simulink model "Racing_Mode"  (R2017b)
settings: Solver=FixedStepAuto  StartTime=0.0  StopTime=10.0  RelTol=1e-3
libraries: simulink x1
settings Model: Creator=cspt  LastModifiedBy=joanv
settings RTWCC: SystemTargetFile=irt.tlc  TemplateMakefile=irt_default_tmf  Description=INTECRIO Real-Time Target
settings STFCustomTargetCC: TargetLangStandard=C99 (ISO)  UtilityFuncGeneration=Shared location  SystemTargetFile=irt.tlc
settings GRTTargetCC: UtilityFuncGeneration=Shared location  ParMdlRefBuildCompliant=off  CompOptLevelCompliant=off  ConcurrentExecutionCompliant=off  CombineOutputUpdateFcns=off  MatFileLogging=off  CPPClassGenCompliant=off  GRTInterface=on  UseToolchainInfoCompliant=off  GenerateASAP2=on

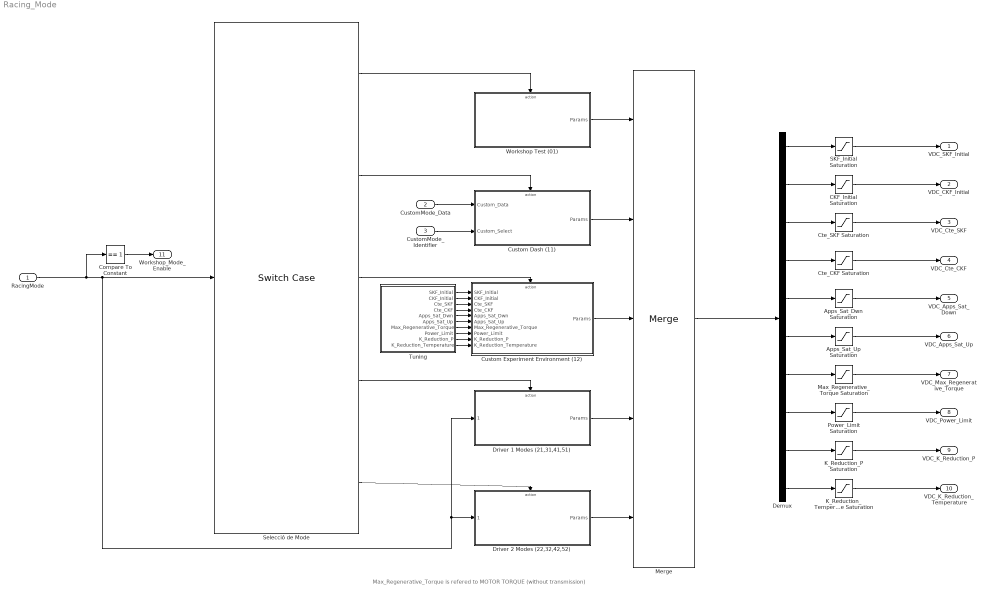
== system Racing_Mode ==
  note: Max_Regenerative_Torque is refered to MOTOR TORQUE (without transmission)
  RacingMode : Inport  OutDataTypeStr=uint8
  CustomMode_Data : Inport  Port=2
  CustomMode_Identifier : Inport  Port=3
  Apps_Sat_Dwn Saturation : Saturate  LowerLimit=0
  Apps_Sat_Up Saturation : Saturate  UpperLimit=1  LowerLimit=0
  CKF_Initial Saturation : Saturate  UpperLimit=0.9  LowerLimit=0
  Compare To Constant : simulink/Logic and Bit Operations/Compare To Constant  relop===  const=1  OutDataTypeStr=boolean
  Cte_CKF Saturation : Saturate  UpperLimit=1  LowerLimit=0
  Cte_SKF Saturation : Saturate  UpperLimit=1  LowerLimit=0
  Custom Dash (11) : Subsystem  TreatAsAtomicUnit=on
  Custom Experiment Environment (12) : Subsystem  TreatAsAtomicUnit=on
  Demux : Demux  Outputs=10
  Driver 1 Modes (21,31,41,51) : Subsystem  TreatAsAtomicUnit=on
  Driver 2 Modes (22,32,42,52) : Subsystem  TreatAsAtomicUnit=on
  K_Reduction_P Saturation : Saturate  UpperLimit=1  LowerLimit=0
  K_Reduction_Temperature Saturation : Saturate  UpperLimit=1  LowerLimit=0
  Max_Regenerative_Torque Saturation : Saturate  UpperLimit=10  LowerLimit=0
  Merge : Merge  Inputs=5
  Power_Limit Saturation : Saturate  UpperLimit=77  LowerLimit=0
  SKF_Initial Saturation : Saturate  UpperLimit=0.9  LowerLimit=0
  Selecció de Mode : SwitchCase  CaseConditions={01, 11, 12, [21,31,41,51], [22,32,42,52]}  ShowDefaultCase=off
  Tuning : Subsystem
  Workshop Test (01) : Subsystem  TreatAsAtomicUnit=on
  VDC_SKF_Initial : Outport
  VDC_CKF_Initial : Outport  Port=2
  VDC_Cte_SKF : Outport  Port=3
  VDC_Cte_CKF : Outport  Port=4
  VDC_Apps_Sat_Down : Outport  Port=5
  VDC_Apps_Sat_Up : Outport  Port=6
  VDC_Max_Regenerative_Torque : Outport  Port=7
  VDC_Power_Limit : Outport  Port=8
  VDC_K_Reduction_P : Outport  Port=9
  VDC_K_Reduction_Temperature : Outport  Port=10
  Workshop_Mode_Enable : Outport  Port=11
  wires:
  RacingMode/1 -> Compare To Constant/1, Driver 2 Modes (22,32,42,52)/1(" "), Driver 1 Modes (21,31,41,51)/1(" "), Selecció de Mode/1
  CKF_Initial Saturation/1 -> VDC_CKF_Initial/1
  Demux/6 -> Apps_Sat_Up Saturation/1
  Demux/3 -> Cte_SKF Saturation/1
  Demux/2 -> CKF_Initial Saturation/1
  Power_Limit Saturation/1 -> VDC_Power_Limit/1
  Apps_Sat_Up Saturation/1 -> VDC_Apps_Sat_Up/1
  Merge/1 -> Demux/1
  CustomMode_Data/1 -> Custom Dash (11)/1(Custom_Data)
  Tuning/7(Max_Regenerative_Torque) -> Custom Experiment Environment (12)/7(Max_Regenerative_Torque)
  Custom Experiment Environment (12)/1(Params) -> Merge/3
  Tuning/9(K_Reduction_P) -> Custom Experiment Environment (12)/9(K_Reduction_P)
  Demux/8 -> Power_Limit Saturation/1
  Tuning/8(Power_Limit) -> Custom Experiment Environment (12)/8(Power_Limit)
  Tuning/4(Cte_CKF) -> Custom Experiment Environment (12)/4(Cte_CKF)
  Selecció de Mode/4 -> Driver 1 Modes (21,31,41,51)/Action
  Demux/4 -> Cte_CKF Saturation/1
  K_Reduction_Temperature Saturation/1 -> VDC_K_Reduction_Temperature/1
  Selecció de Mode/2 -> Custom Dash (11)/Action
  Selecció de Mode/1 -> Workshop Test (01)/Action
  Demux/9 -> K_Reduction_P Saturation/1
  Demux/10 -> K_Reduction_Temperature Saturation/1
  Workshop Test (01)/1(Params) -> Merge/1
  Tuning/5(Apps_Sat_Dwn) -> Custom Experiment Environment (12)/5(Apps_Sat_Dwn)
  Selecció de Mode/5 -> Driver 2 Modes (22,32,42,52)/Action
  Max_Regenerative_Torque Saturation/1 -> VDC_Max_Regenerative_Torque/1
  Cte_CKF Saturation/1 -> VDC_Cte_CKF/1
  Driver 2 Modes (22,32,42,52)/1(Params) -> Merge/5
  Apps_Sat_Dwn Saturation/1 -> VDC_Apps_Sat_Down/1
  Tuning/3(Cte_SKF) -> Custom Experiment Environment (12)/3(Cte_SKF)
  Cte_SKF Saturation/1 -> VDC_Cte_SKF/1
  Tuning/6(Apps_Sat_Up) -> Custom Experiment Environment (12)/6(Apps_Sat_Up)
  Tuning/2(CKF_Initial) -> Custom Experiment Environment (12)/2(CKF_Initial)
  Demux/1 -> SKF_Initial Saturation/1
  K_Reduction_P Saturation/1 -> VDC_K_Reduction_P/1
  Custom Dash (11)/1(Params) -> Merge/2
  Demux/7 -> Max_Regenerative_Torque Saturation/1
  Selecció de Mode/3 -> Custom Experiment Environment (12)/Action
  Tuning/10(K_Reduction_Temperature) -> Custom Experiment Environment (12)/10(K_Reduction_Temperature)
  Demux/5 -> Apps_Sat_Dwn Saturation/1
  SKF_Initial Saturation/1 -> VDC_SKF_Initial/1
  Tuning/1(SKF_Initial) -> Custom Experiment Environment (12)/1(SKF_Initial)
  Driver 1 Modes (21,31,41,51)/1(Params) -> Merge/4
  CustomMode_Identifier/1 -> Custom Dash (11)/2(Custom_Select)
  Compare To Constant/1 -> Workshop_Mode_Enable/1

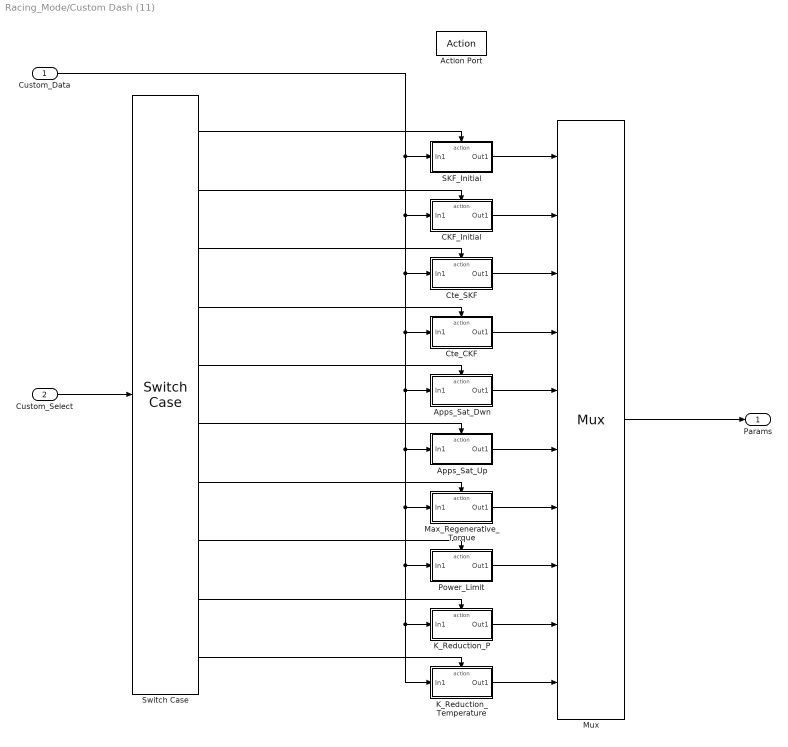
== system Racing_Mode/Custom Dash (11) ==
  Custom_Data : Inport
  Custom_Select : Inport  Port=2
  Action Port : ActionPort  ActionType=case
  Apps_Sat_Dwn : Subsystem  TreatAsAtomicUnit=on
  Apps_Sat_Up : Subsystem  TreatAsAtomicUnit=on
  CKF_Initial : Subsystem  TreatAsAtomicUnit=on
  Cte_CKF : Subsystem  TreatAsAtomicUnit=on
  Cte_SKF : Subsystem  TreatAsAtomicUnit=on
  K_Reduction_P : Subsystem  TreatAsAtomicUnit=on
  K_Reduction_Temperature : Subsystem  TreatAsAtomicUnit=on
  Max_Regenerative_Torque : Subsystem  TreatAsAtomicUnit=on
  Mux : Mux  Inputs=10
  Power_Limit : Subsystem  TreatAsAtomicUnit=on
  SKF_Initial : Subsystem  TreatAsAtomicUnit=on
  Switch Case : SwitchCase  CaseConditions={1,2,3,4,5,6,7,8,9,10}  ShowDefaultCase=off
  Params : Outport
  wires:
  Custom_Select/1 -> Switch Case/1
  Custom_Data/1 -> K_Reduction_Temperature/1(In1), K_Reduction_P/1(In1), Power_Limit/1(In1), Max_Regenerative_Torque/1(In1), Apps_Sat_Up/1(In1), Apps_Sat_Dwn/1(In1), Cte_CKF/1(In1), Cte_SKF/1(In1), CKF_Initial/1(In1), SKF_Initial/1(In1)
  Switch Case/1 -> SKF_Initial/Action
  SKF_Initial/1(Out1) -> Mux/1
  Mux/1 -> Params/1
  CKF_Initial/1(Out1) -> Mux/2
  Cte_SKF/1(Out1) -> Mux/3
  Cte_CKF/1(Out1) -> Mux/4
  Apps_Sat_Dwn/1(Out1) -> Mux/5
  Apps_Sat_Up/1(Out1) -> Mux/6
  Max_Regenerative_Torque/1(Out1) -> Mux/7
  Power_Limit/1(Out1) -> Mux/8
  K_Reduction_P/1(Out1) -> Mux/9
  K_Reduction_Temperature/1(Out1) -> Mux/10
  Switch Case/2 -> CKF_Initial/Action
  Switch Case/3 -> Cte_SKF/Action
  Switch Case/4 -> Cte_CKF/Action
  Switch Case/5 -> Apps_Sat_Dwn/Action
  Switch Case/6 -> Apps_Sat_Up/Action
  Switch Case/7 -> Max_Regenerative_Torque/Action
  Switch Case/8 -> Power_Limit/Action
  Switch Case/9 -> K_Reduction_P/Action
  Switch Case/10 -> K_Reduction_Temperature/Action

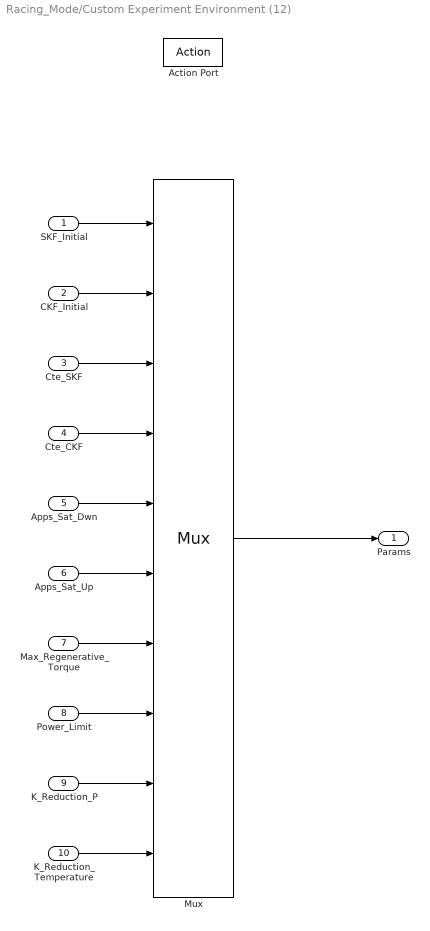
== system Racing_Mode/Custom Experiment Environment (12) ==
  SKF_Initial : Inport
  CKF_Initial : Inport  Port=2
  Cte_SKF : Inport  Port=3
  Cte_CKF : Inport  Port=4
  Apps_Sat_Dwn : Inport  Port=5
  Apps_Sat_Up : Inport  Port=6
  Max_Regenerative_Torque : Inport  Port=7
  Power_Limit : Inport  Port=8
  K_Reduction_P : Inport  Port=9
  K_Reduction_Temperature : Inport  Port=10
  Action Port : ActionPort  ActionType=case
  Mux : Mux  Inputs=10
  Params : Outport
  wires:
  Mux/1 -> Params/1
  K_Reduction_Temperature/1 -> Mux/10
  K_Reduction_P/1 -> Mux/9
  Power_Limit/1 -> Mux/8
  Max_Regenerative_Torque/1 -> Mux/7
  Apps_Sat_Up/1 -> Mux/6
  Apps_Sat_Dwn/1 -> Mux/5
  Cte_CKF/1 -> Mux/4
  Cte_SKF/1 -> Mux/3
  CKF_Initial/1 -> Mux/2
  SKF_Initial/1 -> Mux/1

== system Racing_Mode/Driver 1 Modes (21,31,41,51) ==
  " " : Inport  OutDataTypeStr=uint8
  Action Port : ActionPort  ActionType=case
  "Acceleration (2). Driver 1 (1) " : Subsystem  TreatAsAtomicUnit=on
  AutoX (4). Driver 1 (1) : Subsystem  TreatAsAtomicUnit=on
  Endurance (5). Driver 1 (1) : Subsystem  TreatAsAtomicUnit=on
  Merge : Merge  Inputs=4
  Selecció de Mode : SwitchCase  CaseConditions={21,31,41,51}  ShowDefaultCase=off
  Skidpad (3). Driver 1 (1) : Subsystem  TreatAsAtomicUnit=on
  Params : Outport
  wires:
  Merge/1 -> Params/1
  " "/1 -> Selecció de Mode/1
  Selecció de Mode/4 -> Endurance (5). Driver 1 (1)/Action
  Selecció de Mode/3 -> AutoX (4). Driver 1 (1)/Action
  Selecció de Mode/2 -> Skidpad (3). Driver 1 (1)/Action
  Selecció de Mode/1 -> "Acceleration (2). Driver 1 (1) "/Action
  "Acceleration (2). Driver 1 (1) "/1(Params) -> Merge/1
  Skidpad (3). Driver 1 (1)/1(Params) -> Merge/2
  AutoX (4). Driver 1 (1)/1(Params) -> Merge/3
  Endurance (5). Driver 1 (1)/1(Params) -> Merge/4

== system Racing_Mode/Driver 2 Modes (22,32,42,52) ==
  " " : Inport  OutDataTypeStr=uint8
  Action Port : ActionPort  ActionType=case
  "Acceleration (2). Driver 2 (2) " : Subsystem  TreatAsAtomicUnit=on
  AutoX (4). Driver 2 (2) : Subsystem  TreatAsAtomicUnit=on
  Endurance (5). Driver 2 (2) : Subsystem  TreatAsAtomicUnit=on
  Merge : Merge  Inputs=4
  Selecció de Mode : SwitchCase  CaseConditions={22,32,42,52}  ShowDefaultCase=off
  Skidpad (3). Driver 2 (2) : Subsystem  TreatAsAtomicUnit=on
  Params : Outport
  wires:
  Merge/1 -> Params/1
  " "/1 -> Selecció de Mode/1
  "Acceleration (2). Driver 2 (2) "/1(Params) -> Merge/1
  Skidpad (3). Driver 2 (2)/1(Params) -> Merge/2
  AutoX (4). Driver 2 (2)/1(Params) -> Merge/3
  Endurance (5). Driver 2 (2)/1(Params) -> Merge/4
  Selecció de Mode/4 -> Endurance (5). Driver 2 (2)/Action
  Selecció de Mode/3 -> AutoX (4). Driver 2 (2)/Action
  Selecció de Mode/2 -> Skidpad (3). Driver 2 (2)/Action
  Selecció de Mode/1 -> "Acceleration (2). Driver 2 (2) "/Action

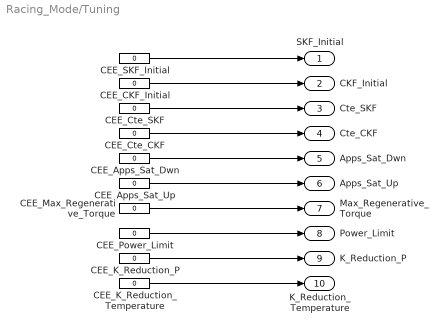
== system Racing_Mode/Tuning ==
  CEE_Apps_Sat_Dwn : Constant  Value=0
  CEE_Apps_Sat_Up : Constant  Value=0
  CEE_CKF_Initial : Constant  Value=0
  CEE_Cte_CKF : Constant  Value=0
  CEE_Cte_SKF : Constant  Value=0
  CEE_K_Reduction_P : Constant  Value=0
  CEE_K_Reduction_Temperature : Constant  Value=0
  CEE_Max_Regenerative_Torque : Constant  Value=0
  CEE_Power_Limit : Constant  Value=0
  CEE_SKF_Initial : Constant  Value=0
  SKF_Initial : Outport
  CKF_Initial : Outport  Port=2
  Cte_SKF : Outport  Port=3
  Cte_CKF : Outport  Port=4
  Apps_Sat_Dwn : Outport  Port=5
  Apps_Sat_Up : Outport  Port=6
  Max_Regenerative_Torque : Outport  Port=7
  Power_Limit : Outport  Port=8
  K_Reduction_P : Outport  Port=9
  K_Reduction_Temperature : Outport  Port=10
  wires:
  CEE_Cte_SKF/1 -> Cte_SKF/1
  CEE_CKF_Initial/1 -> CKF_Initial/1
  CEE_Apps_Sat_Dwn/1 -> Apps_Sat_Dwn/1
  CEE_SKF_Initial/1 -> SKF_Initial/1
  CEE_Max_Regenerative_Torque/1 -> Max_Regenerative_Torque/1
  CEE_Power_Limit/1 -> Power_Limit/1
  CEE_K_Reduction_P/1 -> K_Reduction_P/1
  CEE_K_Reduction_Temperature/1 -> K_Reduction_Temperature/1
  CEE_Apps_Sat_Up/1 -> Apps_Sat_Up/1
  CEE_Cte_CKF/1 -> Cte_CKF/1

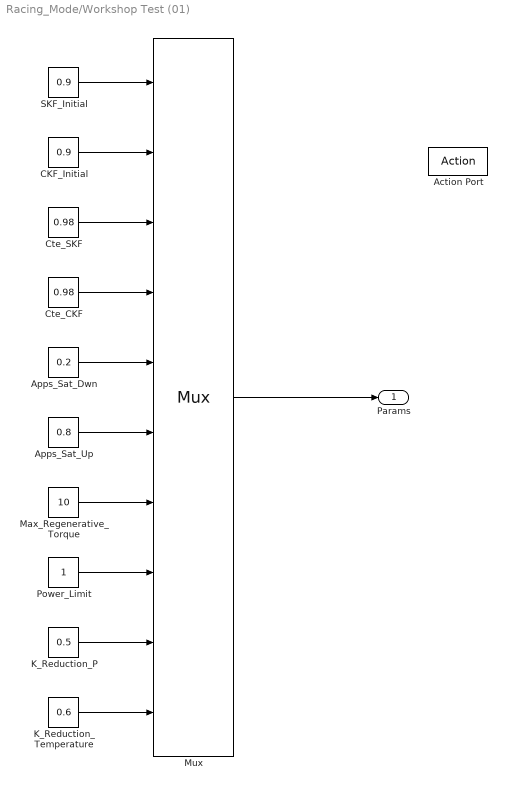
== system Racing_Mode/Workshop Test (01) ==
  Action Port : ActionPort  ActionType=case
  Apps_Sat_Dwn : Constant  Value=0.2
  Apps_Sat_Up : Constant  Value=0.8
  CKF_Initial : Constant  Value=0.9
  Cte_CKF : Constant  Value=0.98
  Cte_SKF : Constant  Value=0.98
  K_Reduction_P : Constant  Value=0.5
  K_Reduction_Temperature : Constant  Value=0.6
  Max_Regenerative_Torque : Constant  Value=10
  Mux : Mux  Inputs=10
  Power_Limit : Constant
  SKF_Initial : Constant  Value=0.9
  Params : Outport
  wires:
  Mux/1 -> Params/1
  SKF_Initial/1 -> Mux/1
  Cte_SKF/1 -> Mux/3
  CKF_Initial/1 -> Mux/2
  Cte_CKF/1 -> Mux/4
  Apps_Sat_Dwn/1 -> Mux/5
  Apps_Sat_Up/1 -> Mux/6
  K_Reduction_Temperature/1 -> Mux/10
  K_Reduction_P/1 -> Mux/9
  Power_Limit/1 -> Mux/8
  Max_Regenerative_Torque/1 -> Mux/7

== system Racing_Mode/Custom Dash (11)/Apps_Sat_Dwn ==
  In1 : Inport
  Action Port : ActionPort  ActionType=case
  Gain : Gain  Gain=1/100
  Out1 : Outport
  wires:
  In1/1 -> Gain/1
  Gain/1 -> Out1/1

== system Racing_Mode/Custom Dash (11)/Apps_Sat_Up ==
  In1 : Inport
  Action Port : ActionPort  ActionType=case
  Gain : Gain  Gain=1/100
  Out1 : Outport
  wires:
  In1/1 -> Gain/1
  Gain/1 -> Out1/1

== system Racing_Mode/Custom Dash (11)/CKF_Initial ==
  In1 : Inport
  Action Port : ActionPort  ActionType=case
  Gain : Gain  Gain=1/1000
  Out1 : Outport
  wires:
  In1/1 -> Gain/1
  Gain/1 -> Out1/1

== system Racing_Mode/Custom Dash (11)/Cte_CKF ==
  In1 : Inport
  Action Port : ActionPort  ActionType=case
  Gain : Gain  Gain=1/1000
  Out1 : Outport
  wires:
  In1/1 -> Gain/1
  Gain/1 -> Out1/1

== system Racing_Mode/Custom Dash (11)/Cte_SKF ==
  In1 : Inport
  Action Port : ActionPort  ActionType=case
  Gain : Gain  Gain=1/1000
  Out1 : Outport
  wires:
  In1/1 -> Gain/1
  Gain/1 -> Out1/1

== system Racing_Mode/Custom Dash (11)/K_Reduction_P ==
  In1 : Inport
  Action Port : ActionPort  ActionType=case
  Gain : Gain  Gain=1/100
  Out1 : Outport
  wires:
  In1/1 -> Gain/1
  Gain/1 -> Out1/1

== system Racing_Mode/Custom Dash (11)/K_Reduction_Temperature ==
  In1 : Inport
  Action Port : ActionPort  ActionType=case
  Gain : Gain  Gain=1/100
  Out1 : Outport
  wires:
  In1/1 -> Gain/1
  Gain/1 -> Out1/1

== system Racing_Mode/Custom Dash (11)/Max_Regenerative_Torque ==
  In1 : Inport
  Action Port : ActionPort  ActionType=case
  Out1 : Outport
  wires:
  In1/1 -> Out1/1

== system Racing_Mode/Custom Dash (11)/Power_Limit ==
  In1 : Inport
  Action Port : ActionPort  ActionType=case
  Out1 : Outport
  wires:
  In1/1 -> Out1/1

== system Racing_Mode/Custom Dash (11)/SKF_Initial ==
  In1 : Inport
  Action Port : ActionPort  ActionType=case
  Gain : Gain  Gain=1/1000
  Out1 : Outport
  wires:
  In1/1 -> Gain/1
  Gain/1 -> Out1/1

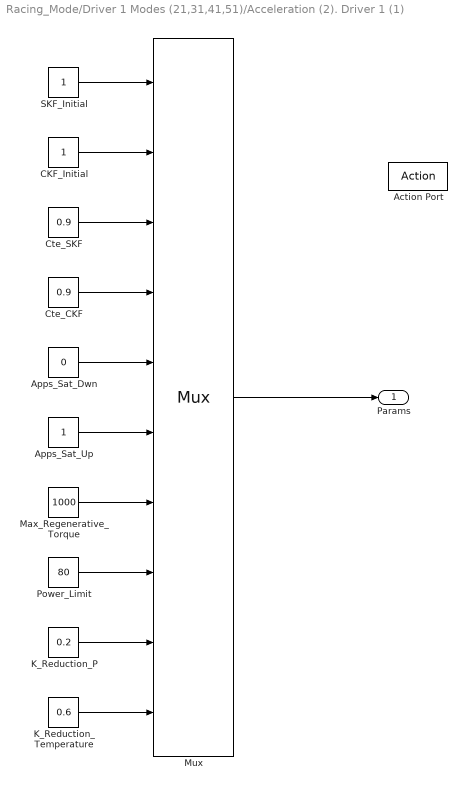
== system Racing_Mode/Driver 1 Modes (21,31,41,51)/Acceleration (2). Driver 1 (1)  ==
  Action Port : ActionPort  ActionType=case
  Apps_Sat_Dwn : Constant  Value=0
  Apps_Sat_Up : Constant
  CKF_Initial : Constant
  Cte_CKF : Constant  Value=0.9
  Cte_SKF : Constant  Value=0.9
  K_Reduction_P : Constant  Value=0.2
  K_Reduction_Temperature : Constant  Value=0.6
  Max_Regenerative_Torque : Constant  Value=1000
  Mux : Mux  Inputs=10
  Power_Limit : Constant  Value=80
  SKF_Initial : Constant
  Params : Outport
  wires:
  Mux/1 -> Params/1
  SKF_Initial/1 -> Mux/1
  Cte_SKF/1 -> Mux/3
  CKF_Initial/1 -> Mux/2
  Cte_CKF/1 -> Mux/4
  Apps_Sat_Dwn/1 -> Mux/5
  Apps_Sat_Up/1 -> Mux/6
  K_Reduction_Temperature/1 -> Mux/10
  K_Reduction_P/1 -> Mux/9
  Power_Limit/1 -> Mux/8
  Max_Regenerative_Torque/1 -> Mux/7

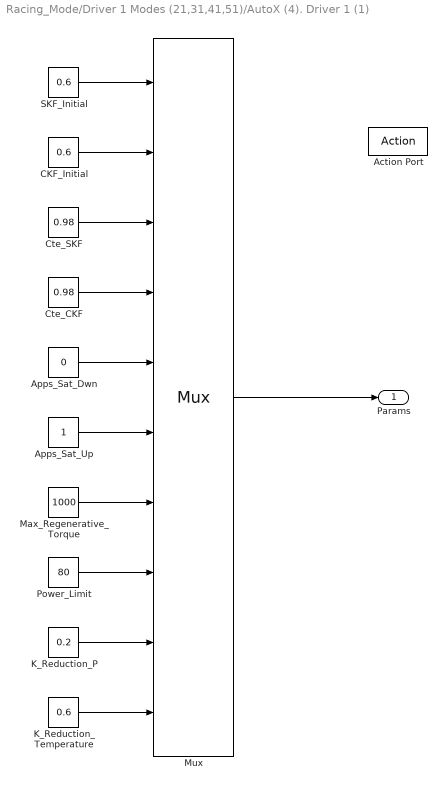
== system Racing_Mode/Driver 1 Modes (21,31,41,51)/AutoX (4). Driver 1 (1) ==
  Action Port : ActionPort  ActionType=case
  Apps_Sat_Dwn : Constant  Value=0
  Apps_Sat_Up : Constant
  CKF_Initial : Constant  Value=0.6
  Cte_CKF : Constant  Value=0.98
  Cte_SKF : Constant  Value=0.98
  K_Reduction_P : Constant  Value=0.2
  K_Reduction_Temperature : Constant  Value=0.6
  Max_Regenerative_Torque : Constant  Value=1000
  Mux : Mux  Inputs=10
  Power_Limit : Constant  Value=80
  SKF_Initial : Constant  Value=0.6
  Params : Outport
  wires:
  Mux/1 -> Params/1
  SKF_Initial/1 -> Mux/1
  Cte_SKF/1 -> Mux/3
  CKF_Initial/1 -> Mux/2
  Cte_CKF/1 -> Mux/4
  Apps_Sat_Dwn/1 -> Mux/5
  Apps_Sat_Up/1 -> Mux/6
  K_Reduction_Temperature/1 -> Mux/10
  K_Reduction_P/1 -> Mux/9
  Power_Limit/1 -> Mux/8
  Max_Regenerative_Torque/1 -> Mux/7

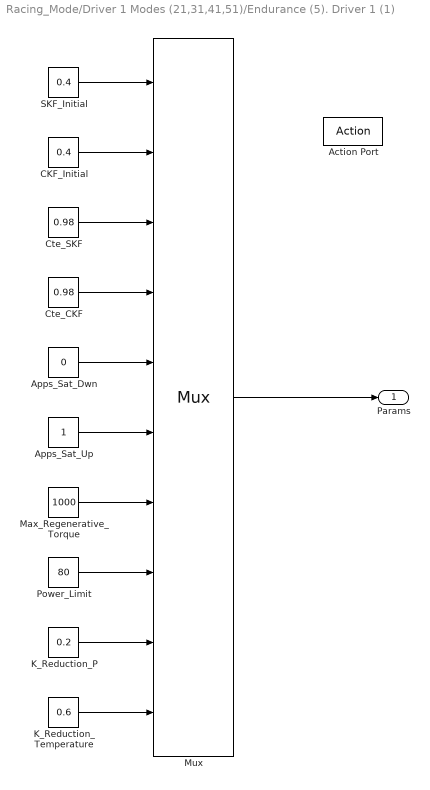
== system Racing_Mode/Driver 1 Modes (21,31,41,51)/Endurance (5). Driver 1 (1) ==
  Action Port : ActionPort  ActionType=case
  Apps_Sat_Dwn : Constant  Value=0
  Apps_Sat_Up : Constant
  CKF_Initial : Constant  Value=0.4
  Cte_CKF : Constant  Value=0.98
  Cte_SKF : Constant  Value=0.98
  K_Reduction_P : Constant  Value=0.2
  K_Reduction_Temperature : Constant  Value=0.6
  Max_Regenerative_Torque : Constant  Value=1000
  Mux : Mux  Inputs=10
  Power_Limit : Constant  Value=80
  SKF_Initial : Constant  Value=0.4
  Params : Outport
  wires:
  Mux/1 -> Params/1
  SKF_Initial/1 -> Mux/1
  Cte_SKF/1 -> Mux/3
  CKF_Initial/1 -> Mux/2
  Cte_CKF/1 -> Mux/4
  Apps_Sat_Dwn/1 -> Mux/5
  Apps_Sat_Up/1 -> Mux/6
  K_Reduction_Temperature/1 -> Mux/10
  K_Reduction_P/1 -> Mux/9
  Power_Limit/1 -> Mux/8
  Max_Regenerative_Torque/1 -> Mux/7

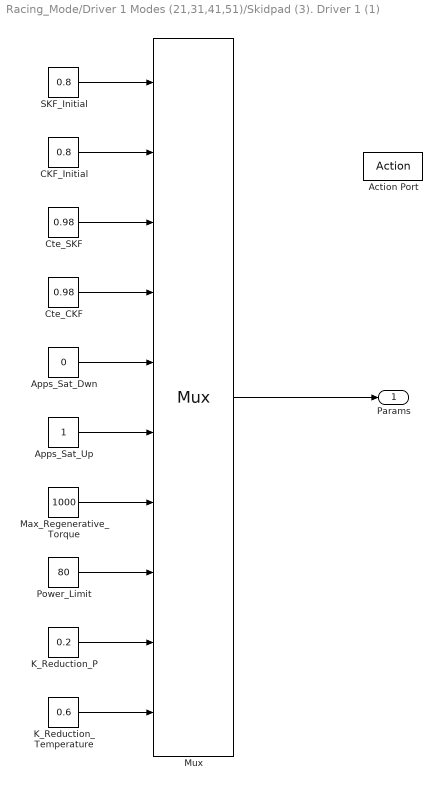
== system Racing_Mode/Driver 1 Modes (21,31,41,51)/Skidpad (3). Driver 1 (1) ==
  Action Port : ActionPort  ActionType=case
  Apps_Sat_Dwn : Constant  Value=0
  Apps_Sat_Up : Constant
  CKF_Initial : Constant  Value=0.8
  Cte_CKF : Constant  Value=0.98
  Cte_SKF : Constant  Value=0.98
  K_Reduction_P : Constant  Value=0.2
  K_Reduction_Temperature : Constant  Value=0.6
  Max_Regenerative_Torque : Constant  Value=1000
  Mux : Mux  Inputs=10
  Power_Limit : Constant  Value=80
  SKF_Initial : Constant  Value=0.8
  Params : Outport
  wires:
  Mux/1 -> Params/1
  SKF_Initial/1 -> Mux/1
  Cte_SKF/1 -> Mux/3
  CKF_Initial/1 -> Mux/2
  Cte_CKF/1 -> Mux/4
  Apps_Sat_Dwn/1 -> Mux/5
  Apps_Sat_Up/1 -> Mux/6
  K_Reduction_Temperature/1 -> Mux/10
  K_Reduction_P/1 -> Mux/9
  Power_Limit/1 -> Mux/8
  Max_Regenerative_Torque/1 -> Mux/7

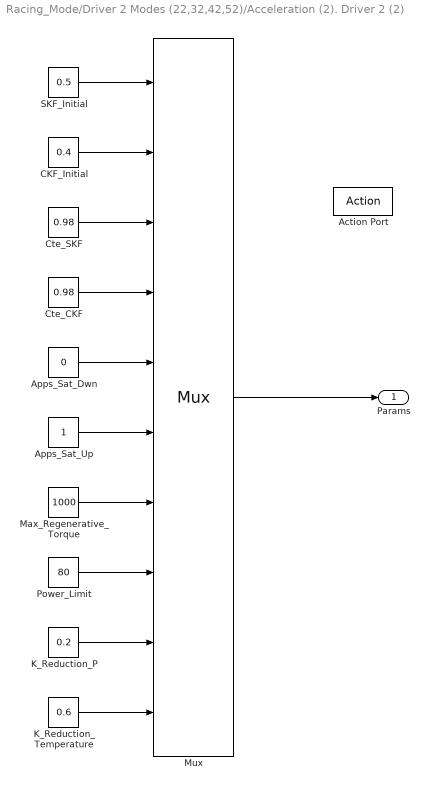
== system Racing_Mode/Driver 2 Modes (22,32,42,52)/Acceleration (2). Driver 2 (2)  ==
  Action Port : ActionPort  ActionType=case
  Apps_Sat_Dwn : Constant  Value=0
  Apps_Sat_Up : Constant
  CKF_Initial : Constant  Value=0.4
  Cte_CKF : Constant  Value=0.98
  Cte_SKF : Constant  Value=0.98
  K_Reduction_P : Constant  Value=0.2
  K_Reduction_Temperature : Constant  Value=0.6
  Max_Regenerative_Torque : Constant  Value=1000
  Mux : Mux  Inputs=10
  Power_Limit : Constant  Value=80
  SKF_Initial : Constant  Value=0.5
  Params : Outport
  wires:
  Mux/1 -> Params/1
  SKF_Initial/1 -> Mux/1
  Cte_SKF/1 -> Mux/3
  CKF_Initial/1 -> Mux/2
  Cte_CKF/1 -> Mux/4
  Apps_Sat_Dwn/1 -> Mux/5
  Apps_Sat_Up/1 -> Mux/6
  K_Reduction_Temperature/1 -> Mux/10
  K_Reduction_P/1 -> Mux/9
  Power_Limit/1 -> Mux/8
  Max_Regenerative_Torque/1 -> Mux/7

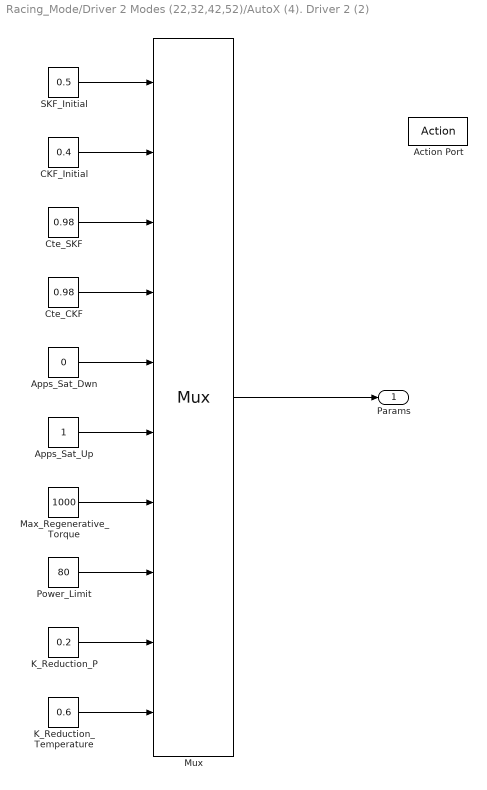
== system Racing_Mode/Driver 2 Modes (22,32,42,52)/AutoX (4). Driver 2 (2) ==
  Action Port : ActionPort  ActionType=case
  Apps_Sat_Dwn : Constant  Value=0
  Apps_Sat_Up : Constant
  CKF_Initial : Constant  Value=0.4
  Cte_CKF : Constant  Value=0.98
  Cte_SKF : Constant  Value=0.98
  K_Reduction_P : Constant  Value=0.2
  K_Reduction_Temperature : Constant  Value=0.6
  Max_Regenerative_Torque : Constant  Value=1000
  Mux : Mux  Inputs=10
  Power_Limit : Constant  Value=80
  SKF_Initial : Constant  Value=0.5
  Params : Outport
  wires:
  Mux/1 -> Params/1
  SKF_Initial/1 -> Mux/1
  Cte_SKF/1 -> Mux/3
  CKF_Initial/1 -> Mux/2
  Cte_CKF/1 -> Mux/4
  Apps_Sat_Dwn/1 -> Mux/5
  Apps_Sat_Up/1 -> Mux/6
  K_Reduction_Temperature/1 -> Mux/10
  K_Reduction_P/1 -> Mux/9
  Power_Limit/1 -> Mux/8
  Max_Regenerative_Torque/1 -> Mux/7

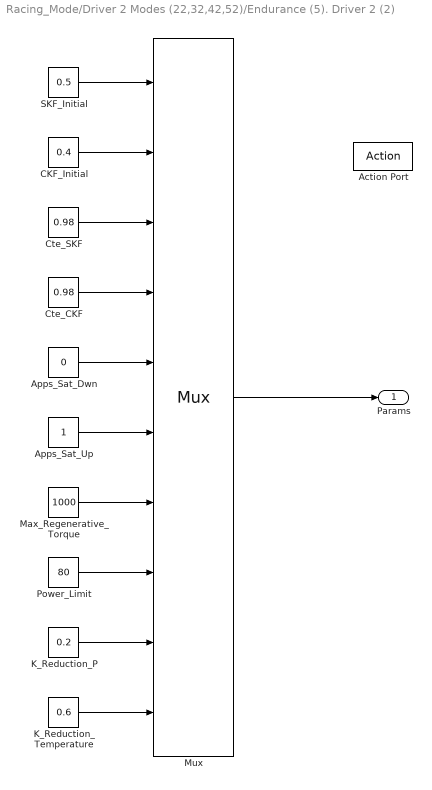
== system Racing_Mode/Driver 2 Modes (22,32,42,52)/Endurance (5). Driver 2 (2) ==
  Action Port : ActionPort  ActionType=case
  Apps_Sat_Dwn : Constant  Value=0
  Apps_Sat_Up : Constant
  CKF_Initial : Constant  Value=0.4
  Cte_CKF : Constant  Value=0.98
  Cte_SKF : Constant  Value=0.98
  K_Reduction_P : Constant  Value=0.2
  K_Reduction_Temperature : Constant  Value=0.6
  Max_Regenerative_Torque : Constant  Value=1000
  Mux : Mux  Inputs=10
  Power_Limit : Constant  Value=80
  SKF_Initial : Constant  Value=0.5
  Params : Outport
  wires:
  Mux/1 -> Params/1
  SKF_Initial/1 -> Mux/1
  Cte_SKF/1 -> Mux/3
  CKF_Initial/1 -> Mux/2
  Cte_CKF/1 -> Mux/4
  Apps_Sat_Dwn/1 -> Mux/5
  Apps_Sat_Up/1 -> Mux/6
  K_Reduction_Temperature/1 -> Mux/10
  K_Reduction_P/1 -> Mux/9
  Power_Limit/1 -> Mux/8
  Max_Regenerative_Torque/1 -> Mux/7

== system Racing_Mode/Driver 2 Modes (22,32,42,52)/Skidpad (3). Driver 2 (2) ==
  Action Port : ActionPort  ActionType=case
  Apps_Sat_Dwn : Constant  Value=0
  Apps_Sat_Up : Constant
  CKF_Initial : Constant  Value=0.4
  Cte_CKF : Constant  Value=0.98
  Cte_SKF : Constant  Value=0.98
  K_Reduction_P : Constant  Value=0.2
  K_Reduction_Temperature : Constant  Value=0.6
  Max_Regenerative_Torque : Constant  Value=1000
  Mux : Mux  Inputs=10
  Power_Limit : Constant  Value=80
  SKF_Initial : Constant  Value=0.5
  Params : Outport
  wires:
  Mux/1 -> Params/1
  SKF_Initial/1 -> Mux/1
  Cte_SKF/1 -> Mux/3
  CKF_Initial/1 -> Mux/2
  Cte_CKF/1 -> Mux/4
  Apps_Sat_Dwn/1 -> Mux/5
  Apps_Sat_Up/1 -> Mux/6
  K_Reduction_Temperature/1 -> Mux/10
  K_Reduction_P/1 -> Mux/9
  Power_Limit/1 -> Mux/8
  Max_Regenerative_Torque/1 -> Mux/7
